simulink model "FaultDetectionModel"  (R2024b)
settings: Solver=VariableStepAuto  StartTime=0.0  StopTime=2  RelTol=1e-3
PostLoadFcn:
  | if ~exist('stdI', 'var')
  |     stdI = 21.8182;
  | end
  | if ~exist('stdV', 'var')
  |     stdV = 5657.2;
  | end
libraries: dspai x1, dspobslib x1
settings Model: Creator=pvenupra  LastModifiedBy=alial
settings DebuggingCC: ParameterPrecisionLossMsg=none

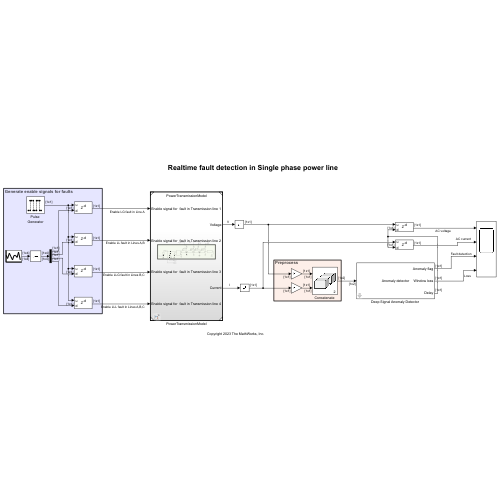
[thumbnail: Simulink's stored preview of the top-level diagram]
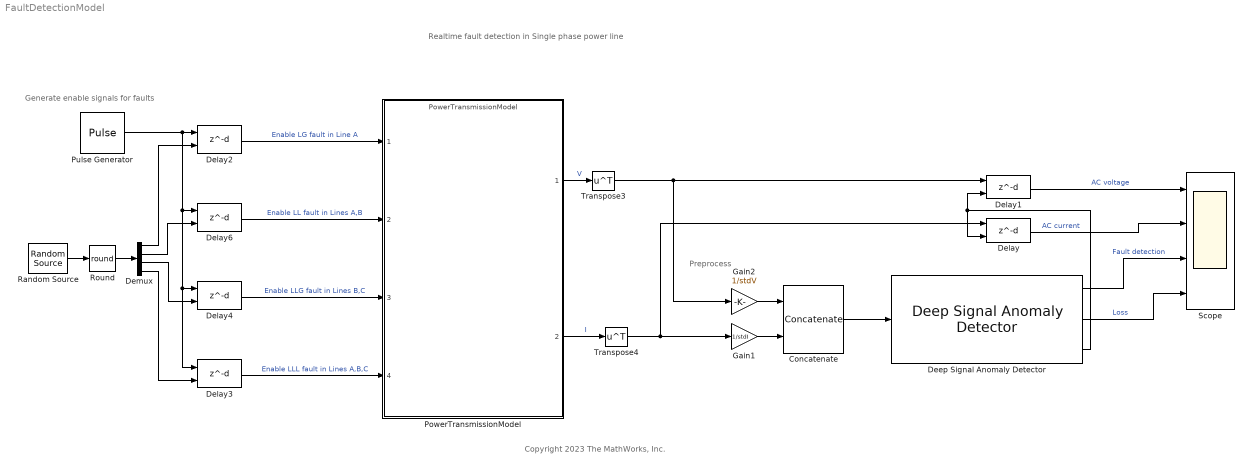
== system FaultDetectionModel ==
  note: Copyright 2023 The MathWorks, Inc.
  note: Preprocess
  note: Realtime fault detection in Single phase power line
  note: Generate enable signals for faults
  "Concatenate " : Concatenate  Mode=Multidimensional array  ConcatenateDimension=2
  "Deep Signal Anomaly Detector " : dspai/Deep Signal Anomaly Detector  DetectorMATFile=singlePhaseFaultDetector.mat  ParameterSource=Read from MAT-file  WindowLength=50  OverlapLength=49  ThresholdSource=Dialog  Threshold=0.032  WindowLossAggregation=Mean  OutputDelay=on
  Delay : Delay  DelayLengthSource=Input port  DelayLengthUpperLimit=200  DiagnosticForDelayLength=Error  InputProcessing=Columns as channels (frame based)
      settings: InputPortMap=u0,p1
  Delay1 : Delay  DelayLengthSource=Input port  DelayLengthUpperLimit=200  DiagnosticForDelayLength=Error  InputProcessing=Columns as channels (frame based)
      settings: InputPortMap=u0,p1
  Delay{2..4,6} (4 alike) : Delay  DelayLengthSource=Input port  DelayLength=1  InputProcessing=Columns as channels (frame based)
      settings: InputPortMap=u0,p1
  Demux : Demux
  Gain1 : Gain  Gain=1/stdI
  Gain2 : Gain  Gain=1/stdV
  PowerTransmissionModel : ModelReference  ModelNameDialog=PowerTransmissionModel.slx  SimulationMode=Normal  ModelReferenceVersion=4.11
  Pulse Generator : DiscretePulseGenerator  Period=1000  PulseWidth=4  SampleTime=.025  VectorParams1D=off
  Random Source : dspobslib/Random Source  SrcType=Uniform  NormMethod=Ziggurat  CltLength=12  MinVal=[0 0.5 1 1.5]*40  MaxVal=[0.4 0.9 1.4 1.9]*40  MeanVal=0  VarVal=1  RepMode=Specify seed  rawSeed=0  IsInherit=off  SampMode=Discrete  SampTime=0.025  SampFrame=1  DataType=Double  OutComplex=Real  OutputFrames=on
  Round : Rounding  Operator=round
  Scope : Scope  NumInputPorts=4
  Transpose3 : Math  Operator=transpose
  Transpose4 : Math  Operator=transpose
  wires:
  "Deep Signal Anomaly Detector "/1 -> Scope/3  "Fault detection"
  "Deep Signal Anomaly Detector "/2 -> Scope/4  "Loss"
  "Concatenate "/1 -> "Deep Signal Anomaly Detector "/1
  Gain2/1 -> "Concatenate "/1
  Gain1/1 -> "Concatenate "/2
  Delay1/1 -> Scope/1  "AC voltage"
  Transpose3/1 -> Delay1/1, Gain2/1
  Transpose4/1 -> Delay/1, Gain1/1
  Random Source/1 -> Round/1
  Delay/1 -> Scope/2  "AC current"
  Pulse Generator/1 -> Delay3/1, Delay4/1, Delay6/1, Delay2/1
  Demux/1 -> Delay2/2
  Demux/2 -> Delay6/2
  Demux/3 -> Delay4/2
  Demux/4 -> Delay3/2
  Round/1 -> Demux/1
  "Deep Signal Anomaly Detector "/3 -> Delay1/2, Delay/2
  PowerTransmissionModel/1 -> Transpose3/1  "V"
  PowerTransmissionModel/2 -> Transpose4/1  "I"
  Delay3/1 -> PowerTransmissionModel/4  "Enable LLL fault in Lines A,B,C"
  Delay4/1 -> PowerTransmissionModel/3  "Enable LLG fault in Lines B,C"
  Delay6/1 -> PowerTransmissionModel/2  "Enable LL fault in Lines A,B"
  Delay2/1 -> PowerTransmissionModel/1  "Enable LG fault in Line A"
